simulink subsystem "PieroCV"  (R2023b)
settings: Solver=VariableStepAuto  StartTime=0.0  StopTime=10.0  RelTol=1e-3
settings Model: Creator=Claudia Ada  LastModifiedBy=pablo

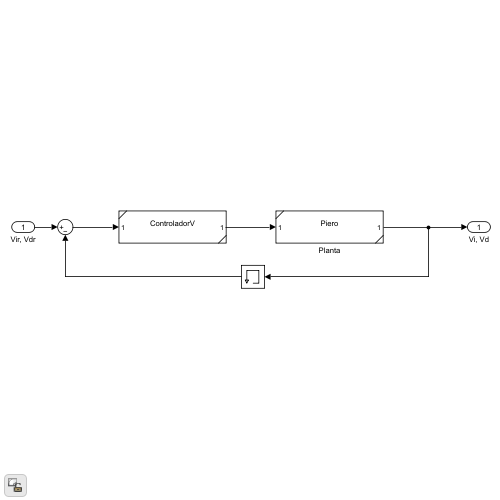
[thumbnail: Simulink's stored preview of the top-level diagram]
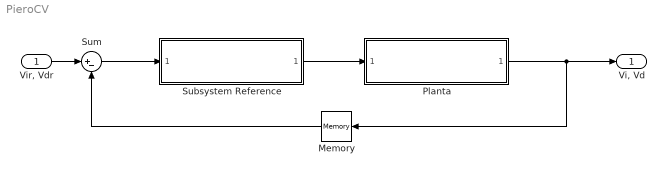
== system PieroCV ==
  "Vir, Vdr" : Inport
  Memory : Memory
  Planta : Subsystem  ReferencedSubsystem=Piero
  Subsystem Reference : Subsystem  ReferencedSubsystem=ControladorV
  Sum : Sum  Inputs=|+-
  "Vi, Vd" : Outport
  wires:
  "Vir, Vdr"/1 -> Sum/1
  Planta/1 -> "Vi, Vd"/1, Memory/1
  Subsystem Reference/1 -> Planta/1
  Sum/1 -> Subsystem Reference/1
  Memory/1 -> Sum/2
